simulink model "feedback_qz1"  (R2015a)
settings: Solver=ode45  StartTime=0.0  StopTime=6  RelTol=1e-3
libraries: cstblocks x3
settings Model: Creator=Kripa95  LastModifiedBy=Kripa95

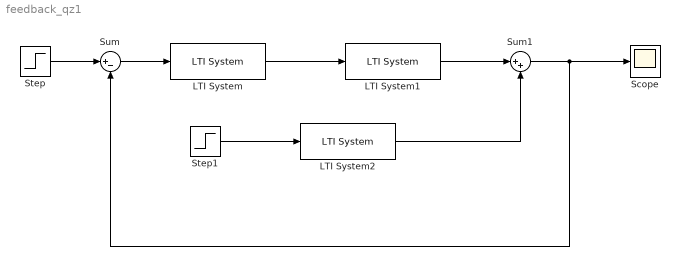
== system feedback_qz1 ==
  LTI System : cstblocks/LTI System  sys=C  IC=[]
  LTI System1 : cstblocks/LTI System  sys=Gvd  IC=[]
  LTI System2 : cstblocks/LTI System  sys=Gvil  IC=[]
  Scope : Scope
      settings: YMin=0.9991  YMax=1.0009
  Step : Step  SampleTime=0
  Step1 : Step  Time=4  SampleTime=0
  Sum : Sum  Inputs=|+-
  Sum1 : Sum  Inputs=|++
  wires:
  Step1/1 -> LTI System2/1
  Step/1 -> Sum/1
  Sum/1 -> LTI System/1
  LTI System/1 -> LTI System1/1
  LTI System1/1 -> Sum1/1
  LTI System2/1 -> Sum1/2
  Sum1/1 -> Sum/2, Scope/1
